simulink model "ICARO3_orientation_controllo_BIPE"  (R2014a)
settings: Solver=FixedStepDiscrete  SolverMode=MultiTasking  StartTime=0.0  StopTime=inf  FixedStep=0.001  RelTol=1e-3
PreLoadFcn:
  | Icaro_path;
  | 
  | load_param;
  | 
  | %override compute_alloc_inside load_param !!!
  | compute_alloc_esa;
  | 
  | load('mag_calib_sim_HIL.mat');
  | 
  | init_adaptive;
InitFcn:
  | %define fast control loop sample time
  | ST = 0.005;
  | 
  | %define filters
  | s = tf('s');
  | 
  | % Derivator (useful in PID controller)
  | D = 0.01*s/(0.01*s+1);
  | 
  | % LP 2nd order filter
  | LP = 42.88/(3.5*s^2 + 19.6*s + 42.88);
  | 
  | %load new DP position controllers
  | progetto_controllo_pos_v1;
undefined symbols (not defined in the file): DiscIntNeverNeededParam, Earth, G, H, INV_PITCH_RANGE, INV_ROLL_RANGE, INV_THROTTLE_RANGE, INV_YAW_RANGE, PITCH_IDX, PITCH_MID, ROLL_IDX, ROLL_MID, RTOL, THROTTLE_DOWN, THROTTLE_IDX, THROTTLE_LOW_THRES, Ts, WGS84, YAW_IDX, YAW_MID
libraries: simulink x15, GPIO_Lib x3, cstblocks x2, aerolibtransform2 x1, STM32_Config_Lib x1
(part 4 of 5)

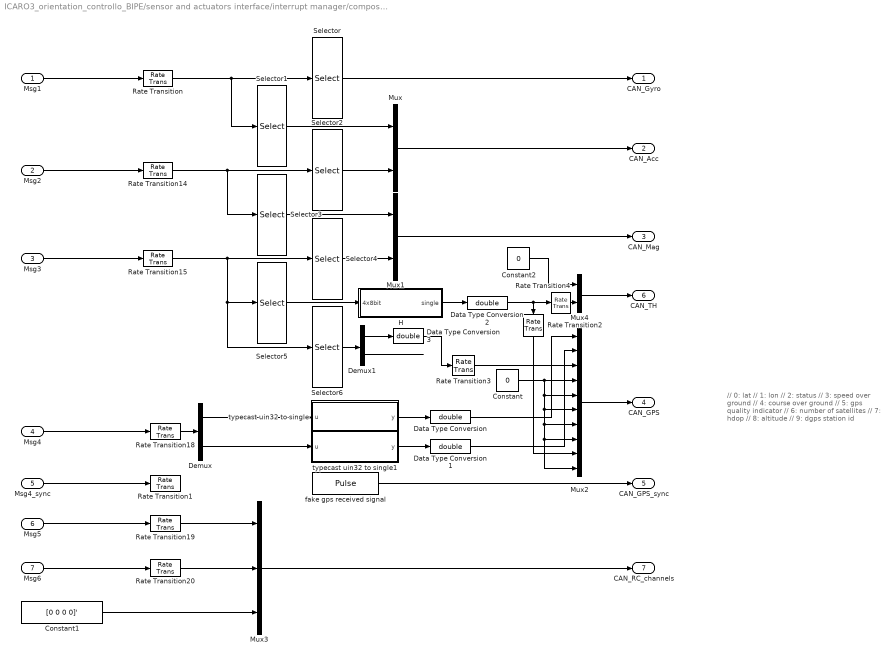
== system ICARO3_orientation_controllo_BIPE/sensor and actuators interface/interrupt manager/compose data from canbus ==
  note: // 0: lat
      |                         // 1: lon
      |                         // 2: status
      |                         // 3: speed over ground
      |                         // 4: course over ground
      |                         // 5: gps quality indicator
      |                         // 6: number of satellites
      |                         // 7: hdop
      |                         // 8: altitude
      |                         // 9: dgps station id
  Msg1 : Inport
  Msg2 : Inport  Port=2
  Msg3 : Inport  Port=3
  Msg4 : Inport  Port=4
  Msg4_sync : Inport  Port=5
  Msg5 : Inport  Port=6
  Msg6 : Inport  Port=7
  Constant : Constant  Value=0
  Constant1 : Constant  Value=[0 0 0 0]'  OutDataTypeStr=uint16
  Constant2 : Constant  Value=0
  Data Type Conversion{,1..3} (4 alike) : DataTypeConversion  OutDataTypeStr=double
  Demux : Demux  Outputs=2
  Demux1 : Demux  Outputs=2
  H : Subsystem
  Mux : Mux  Inputs=2
  Mux1 : Mux  Inputs=2
  Mux2 : Mux  Inputs=10
  Mux3 : Mux  Inputs=3
  Mux4 : Mux  Inputs=2
  Rate Transition{,1,14..15,18..20} (7 alike) : RateTransition  Deterministic=off
  Rate Transition2 : RateTransition
  Rate Transition3 : RateTransition
  Rate Transition4 : RateTransition
  Selector : Selector  InputPortWidth=8  Indices=[1:6]
  Selector1 : Selector  InputPortWidth=8  Indices=[7:8]
  Selector2 : Selector  InputPortWidth=8  Indices=[1:4]
  Selector3 : Selector  InputPortWidth=8  Indices=[5:8]
  Selector4 : Selector  InputPortWidth=8  Indices=[1:2]
  Selector5 : Selector  InputPortWidth=8  Indices=[3:6]
  Selector6 : Selector  InputPortWidth=8  Indices=[7:8]
  fake gps received signal : DiscretePulseGenerator  Period=20  SampleTime=0.01
  typecast uin32 to single : MATLAB Function  TreatAsAtomicUnit=on
      settings: RTWSystemCode=Inline
  typecast uin32 to single1 : MATLAB Function  TreatAsAtomicUnit=on
      settings: RTWSystemCode=Inline
  CAN_Gyro : Outport
  CAN_Acc : Outport  Port=2
  CAN_Mag : Outport  Port=3
  CAN_GPS : Outport  Port=4
  CAN_GPS_sync : Outport  Port=5
  CAN_TH : Outport  Port=6
  CAN_RC_channels : Outport  Port=7
  wires:
  typecast uin32 to single/1(y) -> Data Type Conversion/1
  Demux/1 -> typecast uin32 to single/1(u)
  Demux/2 -> typecast uin32 to single1/1(u)
  fake gps received signal/1 -> CAN_GPS_sync/1
  Data Type Conversion3/1 -> Rate Transition3/1
  Data Type Conversion2/1 -> Rate Transition4/1, Rate Transition2/1
  Data Type Conversion1/1 -> Mux2/2
  Data Type Conversion/1 -> Mux2/1
  Constant2/1 -> Mux4/1
  Rate Transition4/1 -> Mux4/2
  Rate Transition3/1 -> Mux2/3
  Rate Transition2/1 -> Mux2/9
  Mux4/1 -> CAN_TH/1
  Constant1/1 -> Mux3/3
  Mux3/1 -> CAN_RC_channels/1
  Mux2/1 -> CAN_GPS/1
  Demux1/2 -> ?
  Demux1/1 -> Data Type Conversion3/1
  Selector6/1 -> Demux1/1
  Constant/1 -> Mux2/10, Mux2/8, Mux2/7, Mux2/6, Mux2/5, Mux2/4
  Msg4_sync/1 -> Rate Transition1/1
  typecast uin32 to single1/1(y) -> Data Type Conversion1/1
  Rate Transition18/1 -> Demux/1
  H/1(single) -> Data Type Conversion2/1
  Selector5/1 -> H/1(4x8bit)
  Mux1/1 -> CAN_Mag/1
  Selector4/1 -> Mux1/2
  Rate Transition15/1 -> Selector6/1, Selector5/1, Selector4/1
  Selector3/1 -> Mux1/1
  Mux/1 -> CAN_Acc/1
  Selector1/1 -> Mux/1
  Selector2/1 -> Mux/2
  Rate Transition14/1 -> Selector3/1, Selector2/1
  Selector/1 -> CAN_Gyro/1
  Rate Transition/1 -> Selector1/1, Selector/1
  Rate Transition20/1 -> Mux3/2
  Msg6/1 -> Rate Transition20/1
  Rate Transition19/1 -> Mux3/1
  Msg5/1 -> Rate Transition19/1
  Msg4/1 -> Rate Transition18/1
  Msg3/1 -> Rate Transition15/1
  Msg2/1 -> Rate Transition14/1
  Msg1/1 -> Rate Transition/1

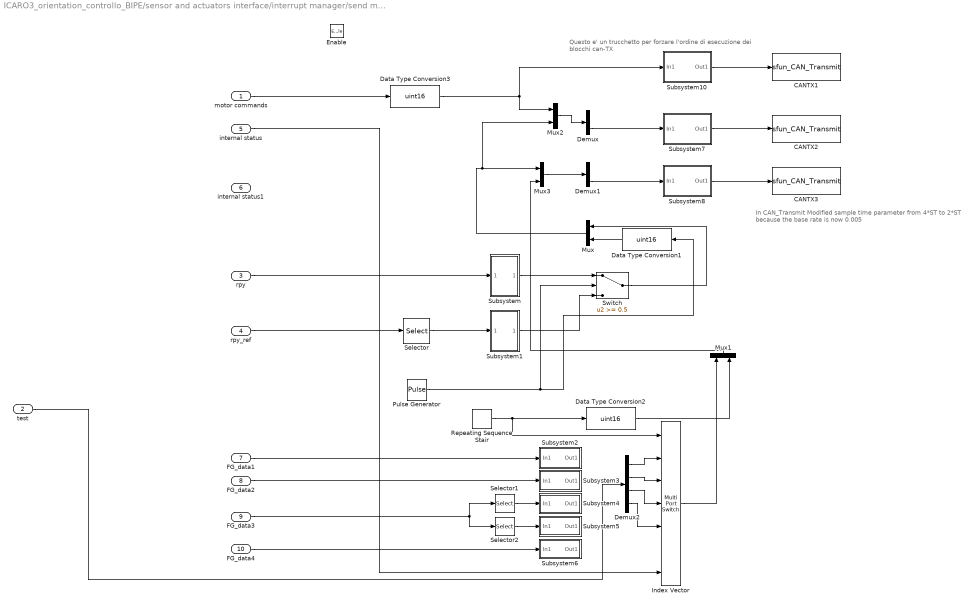
== system ICARO3_orientation_controllo_BIPE/sensor and actuators interface/interrupt manager/send motor commands via canbus ==
  note: In CAN_Transmit Modified sample time parameter from 4*ST to
      | 2*ST because the base rate is now 0.005
  note: Questo e' un trucchetto per forzare l'ordine di esecuzione
      | dei blocchi can-TX
  motor commands : Inport
  test : Inport  Port=2
  rpy : Inport  Port=3
  rpy_ref : Inport  Port=4
  internal status : Inport  Port=5
  internal status1 : Inport  Port=6
  FG_data1 : Inport  Port=7
  FG_data2 : Inport  Port=8
  FG_data3 : Inport  Port=9
  FG_data4 : Inport  Port=10
  Enable : EnablePort
  CANTX1 : S-Function  FunctionName=sfun_CAN_Transmit  Parameters=2*ST,bin2dec('10100001111'),8  EnableBusSupport=off
  CANTX2 : S-Function  FunctionName=sfun_CAN_Transmit  Parameters=2*ST,bin2dec('10100011111'),8  EnableBusSupport=off
  CANTX3 : S-Function  FunctionName=sfun_CAN_Transmit  Parameters=2*ST,bin2dec('10100101111'),8  EnableBusSupport=off
  Data Type Conversion1 : DataTypeConversion  OutDataTypeStr=uint16
  Data Type Conversion2 : DataTypeConversion  OutDataTypeStr=uint16  SampleTime=0.01
  Data Type Conversion3 : DataTypeConversion  OutDataTypeStr=uint16
  Demux : Demux  Outputs=[4 4]
  Demux1 : Demux  Outputs=[4 4]
  Demux2 : Demux  Outputs=[3 3 3 3]
  Index Vector : MultiPortSwitch  DataPortOrder=Zero-based contiguous  Inputs=6  zeroidx=on  SampleTime=0.01
  Mux{,1..3} (4 alike) : Mux  Inputs=2
  Pulse Generator : DiscretePulseGenerator  Period=4  PulseWidth=2  SampleTime=1/100
  Repeating Sequence Stair : simulink/Sources/Repeating Sequence Stair  OutValues=[0 0 1 1 2 2 3 3 4 4 5 5]  tsamp=0.01  OutMin=[]  OutMax=[]  OutDataTypeStr=double  OutputDataTypeScalingMode=double  OutDataType=fixdt(0,8)  ConRadixGroup=Best Precision: Vector-wise  OutScaling=2^-12
  Selector : Selector  InputPortWidth=4  Indices=2:4
  Selector1 : Selector  InputPortWidth=2
  Selector2 : Selector  InputPortWidth=2  Indices=2
  Subsystem : Subsystem
  Subsystem1 : Subsystem
  Subsystem10 : Subsystem
  Subsystem2 : Subsystem
  Subsystem3 : Subsystem
  Subsystem4 : Subsystem
  Subsystem5 : Subsystem
  Subsystem6 : Subsystem
  Subsystem7 : Subsystem
  Subsystem8 : Subsystem
  Switch : Switch  Threshold=0.5
  wires:
  Demux2/4 -> Index Vector/5
  Demux2/3 -> Index Vector/4
  Demux2/1 -> Index Vector/2
  Demux2/2 -> Index Vector/3
  Demux1/2 -> Subsystem8/1(In1)
  test/1 -> Demux2/1
  motor commands/1 -> Data Type Conversion3/1
  Subsystem8/1(Out1) -> CANTX3/1
  rpy_ref/1 -> Selector/1
  Subsystem1/1(Out1) -> Switch/3
  Demux/2 -> Subsystem7/1(In1)
  Subsystem7/1(Out1) -> CANTX2/1
  Subsystem10/1(Out1) -> CANTX1/1
  Data Type Conversion3/1 -> Mux2/1, Subsystem10/1(In1)
  Data Type Conversion2/1 -> Mux1/2
  Data Type Conversion1/1 -> Mux/2
  Repeating Sequence Stair/1 -> Index Vector/1, Data Type Conversion2/1
  FG_data4/1 -> Subsystem6/1(In1)
  FG_data3/1 -> Selector2/1, Selector1/1
  FG_data2/1 -> Subsystem3/1(In1)
  FG_data1/1 -> Subsystem2/1(In1)
  Selector2/1 -> Subsystem5/1(In1)
  Selector1/1 -> Subsystem4/1(In1)
  internal status/1 -> Index Vector/7
  Mux1/1 -> Mux3/2
  Mux3/1 -> Demux1/1
  Mux2/1 -> Demux/1
  Index Vector/1 -> Mux1/1
  Mux/1 -> Mux3/1, Mux2/2
  Selector/1 -> Subsystem1/1(In1)
  Pulse Generator/1 -> Data Type Conversion1/1, Switch/2
  Switch/1 -> Mux/1
  Subsystem/1(Out1) -> Switch/1
  rpy/1 -> Subsystem/1(In1)

== system ICARO3_orientation_controllo_BIPE/ADIS AHRS2/debias ADIS/Acceleration Detrend /Detrend ==
  Input : Inport
  Detrending : Inport  Port=2
  Constant1 : Constant  Value=0
  Subsystem : Subsystem  TreatAsAtomicUnit=on
  Sum1 : Sum  Inputs=|+-  SaturateOnIntegerOverflow=on  InputSameDT=on  OutDataTypeStr=Inherit: Same as first input
  Switch2 : Switch  Threshold=0.5  SaturateOnIntegerOverflow=on  InputSameDT=on
  Detrended Output : Outport
  wires:
  Sum1/1 -> Switch2/3
  Input/1 -> Subsystem/1(In1), Sum1/1
  Constant1/1 -> Switch2/1
  Subsystem/1(Out2) -> Sum1/2
  Detrending/1 -> Subsystem/Enable, Switch2/2
  Switch2/1 -> Detrended Output/1

== system ICARO3_orientation_controllo_BIPE/ADIS AHRS2/debias ADIS/Acceleration Detrend /Detrend1 ==
  Input : Inport
  Detrending : Inport  Port=2
  Constant1 : Constant  Value=0
  Subsystem : Subsystem  TreatAsAtomicUnit=on
  Sum1 : Sum  Inputs=|+-  SaturateOnIntegerOverflow=on  InputSameDT=on  OutDataTypeStr=Inherit: Same as first input
  Switch2 : Switch  Threshold=0.5  SaturateOnIntegerOverflow=on  InputSameDT=on
  Detrended Output : Outport
  wires:
  Switch2/1 -> Detrended Output/1
  Detrending/1 -> Switch2/2, Subsystem/Enable
  Subsystem/1(Out2) -> Sum1/2
  Constant1/1 -> Switch2/1
  Sum1/1 -> Switch2/3
  Input/1 -> Sum1/1, Subsystem/1(In1)

== system ICARO3_orientation_controllo_BIPE/ADIS AHRS2/debias ADIS/Acceleration Detrend /Detrend3 ==
  Input : Inport
  Detrending : Inport  Port=2
  Constant1 : Constant  Value=0
  Constant2 : Constant  Value=9.81
  Subsystem : Subsystem  TreatAsAtomicUnit=on
  Sum1 : Sum  Inputs=|+--  SaturateOnIntegerOverflow=on  InputSameDT=on  OutDataTypeStr=Inherit: Same as first input
  Switch2 : Switch  Threshold=0.5  SaturateOnIntegerOverflow=on  InputSameDT=on
  Detrended Output : Outport
  wires:
  Sum1/1 -> Switch2/3
  Constant2/1 -> Sum1/3
  Input/1 -> Subsystem/1(In1), Sum1/1
  Constant1/1 -> Switch2/1
  Subsystem/1(Out2) -> Sum1/2
  Detrending/1 -> Subsystem/Enable, Switch2/2
  Switch2/1 -> Detrended Output/1

== system ICARO3_orientation_controllo_BIPE/ADIS AHRS2/debias ADIS/Gyros Detrend/Detrend ==
  Input : Inport
  Detrending : Inport  Port=2
  Constant1 : Constant  Value=0
  Subsystem : Subsystem  TreatAsAtomicUnit=on
  Sum1 : Sum  Inputs=|+-  SaturateOnIntegerOverflow=on  InputSameDT=on  OutDataTypeStr=Inherit: Same as first input
  Switch2 : Switch  Threshold=0.5  SaturateOnIntegerOverflow=on  InputSameDT=on
  Detrended Output : Outport
  wires:
  Sum1/1 -> Switch2/3
  Switch2/1 -> Detrended Output/1
  Detrending/1 -> Switch2/2, Subsystem/Enable
  Subsystem/1(Out2) -> Sum1/2
  Constant1/1 -> Switch2/1
  Input/1 -> Sum1/1, Subsystem/1(In1)

== system ICARO3_orientation_controllo_BIPE/ADIS AHRS2/debias ADIS/Gyros Detrend/Detrend1 ==
  Input : Inport
  Detrending : Inport  Port=2
  Constant1 : Constant  Value=0
  Subsystem : Subsystem  TreatAsAtomicUnit=on
  Sum1 : Sum  Inputs=|+-  SaturateOnIntegerOverflow=on  InputSameDT=on  OutDataTypeStr=Inherit: Same as first input
  Switch2 : Switch  Threshold=0.5  SaturateOnIntegerOverflow=on  InputSameDT=on
  Detrended Output : Outport
  wires:
  Sum1/1 -> Switch2/3
  Input/1 -> Subsystem/1(In1), Sum1/1
  Constant1/1 -> Switch2/1
  Subsystem/1(Out2) -> Sum1/2
  Detrending/1 -> Subsystem/Enable, Switch2/2
  Switch2/1 -> Detrended Output/1

== system ICARO3_orientation_controllo_BIPE/ADIS AHRS2/debias ADIS/Gyros Detrend/Detrend2 ==
  Input : Inport
  Detrending : Inport  Port=2
  Constant1 : Constant  Value=0
  Subsystem : Subsystem  TreatAsAtomicUnit=on
  Sum1 : Sum  Inputs=|+-  SaturateOnIntegerOverflow=on  InputSameDT=on  OutDataTypeStr=Inherit: Same as first input
  Switch2 : Switch  Threshold=0.5  SaturateOnIntegerOverflow=on  InputSameDT=on
  Detrended Output : Outport
  wires:
  Sum1/1 -> Switch2/3
  Switch2/1 -> Detrended Output/1
  Detrending/1 -> Switch2/2, Subsystem/Enable
  Subsystem/1(Out2) -> Sum1/2
  Constant1/1 -> Switch2/1
  Input/1 -> Sum1/1, Subsystem/1(In1)

== system ICARO3_orientation_controllo_BIPE/ADIS AHRS2/debias ADIS1/Acceleration Detrend /Detrend ==
  Input : Inport
  Detrending : Inport  Port=2
  Constant1 : Constant  Value=0  OutDataTypeStr=single
  Subsystem : Subsystem  TreatAsAtomicUnit=on
  Sum1 : Sum  Inputs=|+-  SaturateOnIntegerOverflow=on  InputSameDT=on  OutDataTypeStr=Inherit: Same as first input
  Switch2 : Switch  Threshold=0.5  SaturateOnIntegerOverflow=on  InputSameDT=on
  Detrended Output : Outport
  wires:
  Sum1/1 -> Switch2/3
  Input/1 -> Subsystem/1(In1), Sum1/1
  Constant1/1 -> Switch2/1
  Subsystem/1(Out2) -> Sum1/2
  Detrending/1 -> Subsystem/Enable, Switch2/2
  Switch2/1 -> Detrended Output/1

== system ICARO3_orientation_controllo_BIPE/ADIS AHRS2/debias ADIS1/Acceleration Detrend /Detrend1 ==
  Input : Inport
  Detrending : Inport  Port=2
  Constant1 : Constant  Value=0  OutDataTypeStr=single
  Subsystem : Subsystem  TreatAsAtomicUnit=on
  Sum1 : Sum  Inputs=|+-  SaturateOnIntegerOverflow=on  InputSameDT=on  OutDataTypeStr=Inherit: Same as first input
  Switch2 : Switch  Threshold=0.5  SaturateOnIntegerOverflow=on  InputSameDT=on
  Detrended Output : Outport
  wires:
  Switch2/1 -> Detrended Output/1
  Detrending/1 -> Switch2/2, Subsystem/Enable
  Subsystem/1(Out2) -> Sum1/2
  Constant1/1 -> Switch2/1
  Sum1/1 -> Switch2/3
  Input/1 -> Sum1/1, Subsystem/1(In1)

== system ICARO3_orientation_controllo_BIPE/ADIS AHRS2/debias ADIS1/Acceleration Detrend /Detrend3 ==
  Input : Inport
  Detrending : Inport  Port=2
  Constant1 : Constant  Value=0  OutDataTypeStr=single
  Constant2 : Constant  Value=9.81  OutDataTypeStr=single
  Subsystem : Subsystem  TreatAsAtomicUnit=on
  Sum1 : Sum  Inputs=|+--  SaturateOnIntegerOverflow=on  InputSameDT=on  OutDataTypeStr=Inherit: Same as first input
  Switch2 : Switch  Threshold=0.5  SaturateOnIntegerOverflow=on  InputSameDT=on
  Detrended Output : Outport
  wires:
  Sum1/1 -> Switch2/3
  Constant2/1 -> Sum1/3
  Input/1 -> Subsystem/1(In1), Sum1/1
  Constant1/1 -> Switch2/1
  Subsystem/1(Out2) -> Sum1/2
  Switch2/1 -> Detrended Output/1
  Detrending/1 -> Switch2/2, Subsystem/Enable

== system ICARO3_orientation_controllo_BIPE/ADIS AHRS2/debias ADIS1/Acceleration Detrend 1/Detrend ==
  Input : Inport
  Detrending : Inport  Port=2
  Constant1 : Constant  Value=0
  Subsystem : Subsystem  TreatAsAtomicUnit=on
  Sum1 : Sum  Inputs=|+-  SaturateOnIntegerOverflow=on  InputSameDT=on  OutDataTypeStr=Inherit: Same as first input
  Switch2 : Switch  Threshold=0.5  SaturateOnIntegerOverflow=on  InputSameDT=on
  Detrended Output : Outport
  wires:
  Sum1/1 -> Switch2/3
  Input/1 -> Subsystem/1(In1), Sum1/1
  Constant1/1 -> Switch2/1
  Subsystem/1(Out2) -> Sum1/2
  Detrending/1 -> Subsystem/Enable, Switch2/2
  Switch2/1 -> Detrended Output/1

== system ICARO3_orientation_controllo_BIPE/ADIS AHRS2/debias ADIS1/Acceleration Detrend 1/Detrend1 ==
  Input : Inport
  Detrending : Inport  Port=2
  Constant1 : Constant  Value=0
  Subsystem : Subsystem  TreatAsAtomicUnit=on
  Sum1 : Sum  Inputs=|+-  SaturateOnIntegerOverflow=on  InputSameDT=on  OutDataTypeStr=Inherit: Same as first input
  Switch2 : Switch  Threshold=0.5  SaturateOnIntegerOverflow=on  InputSameDT=on
  Detrended Output : Outport
  wires:
  Switch2/1 -> Detrended Output/1
  Detrending/1 -> Switch2/2, Subsystem/Enable
  Subsystem/1(Out2) -> Sum1/2
  Constant1/1 -> Switch2/1
  Sum1/1 -> Switch2/3
  Input/1 -> Sum1/1, Subsystem/1(In1)

== system ICARO3_orientation_controllo_BIPE/ADIS AHRS2/debias ADIS1/Acceleration Detrend 1/Detrend3 ==
  Input : Inport
  Detrending : Inport  Port=2  OutDataTypeStr=single
  Constant1 : Constant  Value=0
  Constant2 : Constant  Value=9.81
  Subsystem : Subsystem  TreatAsAtomicUnit=on
  Sum1 : Sum  Inputs=|+--  SaturateOnIntegerOverflow=on  InputSameDT=on  OutDataTypeStr=Inherit: Same as first input
  Switch2 : Switch  Threshold=0.5  SaturateOnIntegerOverflow=on  InputSameDT=on
  Detrended Output : Outport
  wires:
  Sum1/1 -> Switch2/3
  Constant2/1 -> Sum1/3
  Input/1 -> Subsystem/1(In1), Sum1/1
  Constant1/1 -> Switch2/1
  Subsystem/1(Out2) -> Sum1/2
  Switch2/1 -> Detrended Output/1
  Detrending/1 -> Switch2/2, Subsystem/Enable

== system ICARO3_orientation_controllo_BIPE/ADIS AHRS2/debias ADIS1/Gyros Detrend/Detrend ==
  Input : Inport
  Detrending : Inport  Port=2
  Constant1 : Constant  Value=0
  Data Type Conversion mx3 : DataTypeConversion  OutDataTypeStr=double  RndMeth=Round  SaturateOnIntegerOverflow=on
  Subsystem : Subsystem  TreatAsAtomicUnit=on
  Sum1 : Sum  Inputs=|+-  SaturateOnIntegerOverflow=on  InputSameDT=on  OutDataTypeStr=Inherit: Same as first input
  Switch2 : Switch  Threshold=0.5  SaturateOnIntegerOverflow=on  InputSameDT=on
  Detrended Output : Outport
  wires:
  Switch2/1 -> Detrended Output/1
  Detrending/1 -> Switch2/2, Subsystem/Enable
  Subsystem/1(Out2) -> Sum1/2
  Constant1/1 -> Switch2/1
  Input/1 -> Sum1/1, Subsystem/1(In1)
  Sum1/1 -> Data Type Conversion mx3/1
  Data Type Conversion mx3/1 -> Switch2/3

== system ICARO3_orientation_controllo_BIPE/ADIS AHRS2/debias ADIS1/Gyros Detrend/Detrend1 ==
  Input : Inport
  Detrending : Inport  Port=2
  Constant1 : Constant  Value=0
  Data Type Conversion mx3 : DataTypeConversion  OutDataTypeStr=double  RndMeth=Round  SaturateOnIntegerOverflow=on
  Subsystem : Subsystem  TreatAsAtomicUnit=on
  Sum1 : Sum  Inputs=|+-  SaturateOnIntegerOverflow=on  InputSameDT=on  OutDataTypeStr=Inherit: Same as first input
  Switch2 : Switch  Threshold=0.5  SaturateOnIntegerOverflow=on  InputSameDT=on
  Detrended Output : Outport
  wires:
  Sum1/1 -> Data Type Conversion mx3/1
  Input/1 -> Subsystem/1(In1), Sum1/1
  Constant1/1 -> Switch2/1
  Subsystem/1(Out2) -> Sum1/2
  Detrending/1 -> Subsystem/Enable, Switch2/2
  Switch2/1 -> Detrended Output/1
  Data Type Conversion mx3/1 -> Switch2/3

== system ICARO3_orientation_controllo_BIPE/ADIS AHRS2/debias ADIS1/Gyros Detrend/Detrend2 ==
  Input : Inport
  Detrending : Inport  Port=2
  Constant1 : Constant  Value=0
  Data Type Conversion mx3 : DataTypeConversion  OutDataTypeStr=double  RndMeth=Round  SaturateOnIntegerOverflow=on
  Subsystem : Subsystem  TreatAsAtomicUnit=on
  Sum1 : Sum  Inputs=|+-  SaturateOnIntegerOverflow=on  InputSameDT=on  OutDataTypeStr=Inherit: Same as first input
  Switch2 : Switch  Threshold=0.5  SaturateOnIntegerOverflow=on  InputSameDT=on
  Detrended Output : Outport
  wires:
  Sum1/1 -> Data Type Conversion mx3/1
  Switch2/1 -> Detrended Output/1
  Detrending/1 -> Switch2/2, Subsystem/Enable
  Subsystem/1(Out2) -> Sum1/2
  Constant1/1 -> Switch2/1
  Input/1 -> Sum1/1, Subsystem/1(In1)
  Data Type Conversion mx3/1 -> Switch2/3

== system ICARO3_orientation_controllo_BIPE/SS AHRS/debias SS/Acceleration Detrend /Detrend ==
  Input : Inport
  Detrending : Inport  Port=2
  Constant1 : Constant  Value=0
  Subsystem : Subsystem  TreatAsAtomicUnit=on
  Sum1 : Sum  Inputs=|+-  SaturateOnIntegerOverflow=on  InputSameDT=on  OutDataTypeStr=Inherit: Same as first input
  Switch2 : Switch  Threshold=0.5  SaturateOnIntegerOverflow=on  InputSameDT=on
  Detrended Output : Outport
  wires:
  Switch2/1 -> Detrended Output/1
  Detrending/1 -> Switch2/2, Subsystem/Enable
  Subsystem/1(Out2) -> Sum1/2
  Constant1/1 -> Switch2/1
  Input/1 -> Sum1/1, Subsystem/1(In1)
  Sum1/1 -> Switch2/3

== system ICARO3_orientation_controllo_BIPE/SS AHRS/debias SS/Acceleration Detrend /Detrend1 ==
  Input : Inport
  Detrending : Inport  Port=2
  Constant1 : Constant  Value=0
  Subsystem : Subsystem  TreatAsAtomicUnit=on
  Sum1 : Sum  Inputs=|+-  SaturateOnIntegerOverflow=on  InputSameDT=on  OutDataTypeStr=Inherit: Same as first input
  Switch2 : Switch  Threshold=0.5  SaturateOnIntegerOverflow=on  InputSameDT=on
  Detrended Output : Outport
  wires:
  Input/1 -> Subsystem/1(In1), Sum1/1
  Sum1/1 -> Switch2/3
  Constant1/1 -> Switch2/1
  Subsystem/1(Out2) -> Sum1/2
  Detrending/1 -> Subsystem/Enable, Switch2/2
  Switch2/1 -> Detrended Output/1

== system ICARO3_orientation_controllo_BIPE/SS AHRS/debias SS/Acceleration Detrend /Detrend3 ==
  Input : Inport
  Detrending : Inport  Port=2
  Constant1 : Constant  Value=0
  Constant2 : Constant  Value=9.81
  Subsystem : Subsystem  TreatAsAtomicUnit=on
  Sum1 : Sum  Inputs=|+--  SaturateOnIntegerOverflow=on  InputSameDT=on  OutDataTypeStr=Inherit: Same as first input
  Switch2 : Switch  Threshold=0.5  SaturateOnIntegerOverflow=on  InputSameDT=on
  Detrended Output : Outport
  wires:
  Switch2/1 -> Detrended Output/1
  Detrending/1 -> Switch2/2, Subsystem/Enable
  Subsystem/1(Out2) -> Sum1/2
  Constant1/1 -> Switch2/1
  Input/1 -> Sum1/1, Subsystem/1(In1)
  Constant2/1 -> Sum1/3
  Sum1/1 -> Switch2/3

== system ICARO3_orientation_controllo_BIPE/SS AHRS/debias SS/Gyros Detrend/Detrend ==
  Input : Inport
  Detrending : Inport  Port=2
  Constant1 : Constant  Value=0
  Subsystem : Subsystem  TreatAsAtomicUnit=on
  Sum1 : Sum  Inputs=|+-  SaturateOnIntegerOverflow=on  InputSameDT=on  OutDataTypeStr=Inherit: Same as first input
  Switch2 : Switch  Threshold=0.5  SaturateOnIntegerOverflow=on  InputSameDT=on
  Detrended Output : Outport
  wires:
  Input/1 -> Subsystem/1(In1), Sum1/1
  Constant1/1 -> Switch2/1
  Subsystem/1(Out2) -> Sum1/2
  Detrending/1 -> Subsystem/Enable, Switch2/2
  Switch2/1 -> Detrended Output/1
  Sum1/1 -> Switch2/3

== system ICARO3_orientation_controllo_BIPE/SS AHRS/debias SS/Gyros Detrend/Detrend1 ==
  Input : Inport
  Detrending : Inport  Port=2
  Constant1 : Constant  Value=0
  Subsystem : Subsystem  TreatAsAtomicUnit=on
  Sum1 : Sum  Inputs=|+-  SaturateOnIntegerOverflow=on  InputSameDT=on  OutDataTypeStr=Inherit: Same as first input
  Switch2 : Switch  Threshold=0.5  SaturateOnIntegerOverflow=on  InputSameDT=on
  Detrended Output : Outport
  wires:
  Switch2/1 -> Detrended Output/1
  Detrending/1 -> Switch2/2, Subsystem/Enable
  Subsystem/1(Out2) -> Sum1/2
  Constant1/1 -> Switch2/1
  Input/1 -> Sum1/1, Subsystem/1(In1)
  Sum1/1 -> Switch2/3

== system ICARO3_orientation_controllo_BIPE/SS AHRS/debias SS/Gyros Detrend/Detrend2 ==
  Input : Inport
  Detrending : Inport  Port=2
  Constant1 : Constant  Value=0
  Subsystem : Subsystem  TreatAsAtomicUnit=on
  Sum1 : Sum  Inputs=|+-  SaturateOnIntegerOverflow=on  InputSameDT=on  OutDataTypeStr=Inherit: Same as first input
  Switch2 : Switch  Threshold=0.5  SaturateOnIntegerOverflow=on  InputSameDT=on
  Detrended Output : Outport
  wires:
  Input/1 -> Subsystem/1(In1), Sum1/1
  Constant1/1 -> Switch2/1
  Subsystem/1(Out2) -> Sum1/2
  Detrending/1 -> Subsystem/Enable, Switch2/2
  Switch2/1 -> Detrended Output/1
  Sum1/1 -> Switch2/3

== system ICARO3_orientation_controllo_BIPE/sensor and actuators interface/interrupt manager/Arrange pwms/clock latch ==
  note: NOTE: initial output value of OUTPORT
      | is set to -1000 to ensure that the first computed age
      | at the start of autopilot is at least 1000 !
      | (otherwise it was 0)
  In : Inport
  Enable : EnablePort
  Out : Outport  InitialOutput=-1000
  wires:
  In/1 -> Out/1

== system ICARO3_orientation_controllo_BIPE/sensor and actuators interface/interrupt manager/CANbus data RX/Subsystem1 ==
  In1 : Inport
  Data Type Conversion on i2c mag1 : DataTypeConversion  OutDataTypeStr=uint16
  Demux3 : Demux  Outputs=[ 2 2 2 2]
  MATLAB Function compute gyroxyz1 : MATLAB Function  TreatAsAtomicUnit=on
  MATLAB Function compute gyroxyz2 : MATLAB Function  TreatAsAtomicUnit=on
  MATLAB Function compute gyroxyz3 : MATLAB Function  TreatAsAtomicUnit=on
  MATLAB Function compute gyroxyz5 : MATLAB Function  TreatAsAtomicUnit=on
  Mux : Mux
  Out1 : Outport
  wires:
  MATLAB Function compute gyroxyz5/1(y) -> Mux/1
  Mux/1 -> Out1/1
  MATLAB Function compute gyroxyz3/1(y) -> Mux/4
  MATLAB Function compute gyroxyz1/1(y) -> Mux/2
  Demux3/2 -> MATLAB Function compute gyroxyz1/1(u)
  Demux3/3 -> MATLAB Function compute gyroxyz2/1(u)
  MATLAB Function compute gyroxyz2/1(y) -> Mux/3
  Data Type Conversion on i2c mag1/1 -> Demux3/1
  Demux3/1 -> MATLAB Function compute gyroxyz5/1(u)
  In1/1 -> Data Type Conversion on i2c mag1/1
  Demux3/4 -> MATLAB Function compute gyroxyz3/1(u)

== system ICARO3_orientation_controllo_BIPE/sensor and actuators interface/interrupt manager/CANbus data RX/Subsystem2 ==
  In1 : Inport
  Data Type Conversion on i2c mag1 : DataTypeConversion  OutDataTypeStr=uint32
  Demux3 : Demux  Outputs=[ 4 4]
  MATLAB Function compute gyroxyz1 : MATLAB Function  TreatAsAtomicUnit=on
  MATLAB Function compute gyroxyz5 : MATLAB Function  TreatAsAtomicUnit=on
  Mux : Mux  Inputs=2
  Out1 : Outport
  wires:
  MATLAB Function compute gyroxyz1/1(y) -> Mux/2
  Demux3/2 -> MATLAB Function compute gyroxyz1/1(u)
  Data Type Conversion on i2c mag1/1 -> Demux3/1
  MATLAB Function compute gyroxyz5/1(y) -> Mux/1
  Demux3/1 -> MATLAB Function compute gyroxyz5/1(u)
  In1/1 -> Data Type Conversion on i2c mag1/1
  Mux/1 -> Out1/1

== system ICARO3_orientation_controllo_BIPE/sensor and actuators interface/interrupt manager/CANbus data RX/Subsystem3 ==
  In1 : Inport
  Data Type Conversion on i2c mag1 : DataTypeConversion  OutDataTypeStr=uint16
  Demux3 : Demux  Outputs=[ 2 2 2 2]
  MATLAB Function compute gyroxyz1 : MATLAB Function  TreatAsAtomicUnit=on
  MATLAB Function compute gyroxyz2 : MATLAB Function  TreatAsAtomicUnit=on
  MATLAB Function compute gyroxyz3 : MATLAB Function  TreatAsAtomicUnit=on
  MATLAB Function compute gyroxyz5 : MATLAB Function  TreatAsAtomicUnit=on
  Mux : Mux
  Out1 : Outport
  wires:
  Demux3/4 -> MATLAB Function compute gyroxyz3/1(u)
  In1/1 -> Data Type Conversion on i2c mag1/1
  Demux3/1 -> MATLAB Function compute gyroxyz5/1(u)
  Data Type Conversion on i2c mag1/1 -> Demux3/1
  MATLAB Function compute gyroxyz2/1(y) -> Mux/3
  Demux3/3 -> MATLAB Function compute gyroxyz2/1(u)
  Demux3/2 -> MATLAB Function compute gyroxyz1/1(u)
  MATLAB Function compute gyroxyz1/1(y) -> Mux/2
  MATLAB Function compute gyroxyz3/1(y) -> Mux/4
  Mux/1 -> Out1/1
  MATLAB Function compute gyroxyz5/1(y) -> Mux/1

== matlab function ICARO3_orientation_controllo_BIPE/sensor and actuators interface/interrupt manager/send motor commands via canbus/Subsystem7/MATLAB Function compute gyroxyz1 ==
  settings: updateMethod=DISCRETE  sampleTime=0.01
  data: u input uint16; y output uint8
function y = pack2_8bit(u)

y =uint8([0,0]);
y(1) = bitand(u,255);
y(2) = bitshift(u,-8);

== matlab function ICARO3_orientation_controllo_BIPE/sensor and actuators interface/interrupt manager/send motor commands via canbus/Subsystem7/MATLAB Function compute gyroxyz4 ==
  settings: updateMethod=DISCRETE  sampleTime=0.01
  data: u input uint8; y output uint8
function y = reorder(u)

y=uint8(zeros(1,8));
y(1)=u(1);
y(2)=u(2);
y(3)=u(3);
y(4)=u(4);
y(5)=u(5);
y(6)=u(6);
y(7)=u(7);
y(8)=u(8);

== matlab function ICARO3_orientation_controllo_BIPE/sensor and actuators interface/interrupt manager/send motor commands via canbus/Subsystem8/MATLAB Function compute gyroxyz4 ==
  settings: updateMethod=DISCRETE  sampleTime=0.01
  data: u input uint8; y output uint8
function y = reorder(u)

y=uint8(zeros(1,8));
y(1)=u(1);
y(2)=u(2);
y(3)=u(3);
y(4)=u(4);
y(5)=u(5);
y(6)=u(6);
y(7)=u(7);
y(8)=u(8);

== system ICARO3_orientation_controllo_BIPE/sensor and actuators interface/interrupt manager/compose data from canbus/H ==
  4x8bit : Inport
  " " : ArithShift  BitShiftNumber=24  BitShiftDirection=Left
  "  " : ArithShift  BitShiftNumber=16  BitShiftDirection=Left
  "  2" : ArithShift  BitShiftNumber=8  BitShiftDirection=Left
  Data Type Conversion{7..10} (4 alike) : DataTypeConversion  OutDataTypeStr=uint32
  Demux : Demux
  Sum12 : Sum  Inputs=++++
  typecast uin32 to single : MATLAB Function  TreatAsAtomicUnit=on
      settings: RTWSystemCode=Inline
  single : Outport
  wires:
  4x8bit/1 -> Demux/1
  Demux/4 -> Data Type Conversion10/1
  Demux/3 -> Data Type Conversion7/1
  Demux/2 -> Data Type Conversion9/1
  Demux/1 -> Data Type Conversion8/1
  typecast uin32 to single/1(y) -> single/1
  Sum12/1 -> typecast uin32 to single/1(u)
  " "/1 -> Sum12/1
  Data Type Conversion10/1 -> Sum12/4
  "  2"/1 -> Sum12/3
  "  "/1 -> Sum12/2
  Data Type Conversion7/1 -> "  2"/1
  Data Type Conversion9/1 -> "  "/1
  Data Type Conversion8/1 -> " "/1

== system ICARO3_orientation_controllo_BIPE/sensor and actuators interface/interrupt manager/send motor commands via canbus/Subsystem ==
  In1 : Inport
  Constant : Constant  Value=180
  Data Type Conversion2 : DataTypeConversion  OutDataTypeStr=uint16
  Gain : Gain  Gain=180/pi
  Sum : Sum  Inputs=|++
  Out1 : Outport
  wires:
  In1/1 -> Gain/1
  Data Type Conversion2/1 -> Out1/1
  Sum/1 -> Data Type Conversion2/1
  Constant/1 -> Sum/2
  Gain/1 -> Sum/1

== system ICARO3_orientation_controllo_BIPE/sensor and actuators interface/interrupt manager/send motor commands via canbus/Subsystem1 ==
  In1 : Inport
  Constant : Constant  Value=180
  Data Type Conversion2 : DataTypeConversion  OutDataTypeStr=uint16
  Gain : Gain  Gain=180/pi
  Sum : Sum  Inputs=|++
  Out1 : Outport
  wires:
  Gain/1 -> Sum/1
  Constant/1 -> Sum/2
  Sum/1 -> Data Type Conversion2/1
  Data Type Conversion2/1 -> Out1/1
  In1/1 -> Gain/1

== system ICARO3_orientation_controllo_BIPE/sensor and actuators interface/interrupt manager/send motor commands via canbus/Subsystem10 ==
  In1 : Inport
  Demux3 : Demux  Outputs=[1 1 1 1]
  MATLAB Function compute gyroxyz1 : MATLAB Function  TreatAsAtomicUnit=on
  MATLAB Function compute gyroxyz2 : MATLAB Function  TreatAsAtomicUnit=on
  MATLAB Function compute gyroxyz3 : MATLAB Function  TreatAsAtomicUnit=on
  MATLAB Function compute gyroxyz4 : MATLAB Function  TreatAsAtomicUnit=on
  MATLAB Function compute gyroxyz5 : MATLAB Function  TreatAsAtomicUnit=on
  Mux1 : Mux  Inputs=[2 2 2 2]
  Out1 : Outport
  wires:
  MATLAB Function compute gyroxyz4/1(y) -> Out1/1
  Mux1/1 -> MATLAB Function compute gyroxyz4/1(u)
  MATLAB Function compute gyroxyz5/1(y) -> Mux1/1
  MATLAB Function compute gyroxyz3/1(y) -> Mux1/4
  MATLAB Function compute gyroxyz2/1(y) -> Mux1/3
  MATLAB Function compute gyroxyz1/1(y) -> Mux1/2
  Demux3/2 -> MATLAB Function compute gyroxyz1/1(u)
  Demux3/3 -> MATLAB Function compute gyroxyz2/1(u)
  In1/1 -> Demux3/1
  Demux3/1 -> MATLAB Function compute gyroxyz5/1(u)
  Demux3/4 -> MATLAB Function compute gyroxyz3/1(u)

== system ICARO3_orientation_controllo_BIPE/sensor and actuators interface/interrupt manager/send motor commands via canbus/Subsystem2 ==
  In1 : Inport
  Constant : Constant  Value=2047  SampleTime=0.01
  Data Type Conversion2 : DataTypeConversion  OutDataTypeStr=uint16
  Gain : Gain  Gain=100
  Sum : Sum  Inputs=|++
  Out1 : Outport
  wires:
  Gain/1 -> Sum/1
  Constant/1 -> Sum/2
  Sum/1 -> Data Type Conversion2/1
  Data Type Conversion2/1 -> Out1/1
  In1/1 -> Gain/1

== system ICARO3_orientation_controllo_BIPE/sensor and actuators interface/interrupt manager/send motor commands via canbus/Subsystem3 ==
  In1 : Inport
  Constant : Constant  Value=2047  SampleTime=0.01
  Data Type Conversion2 : DataTypeConversion  OutDataTypeStr=uint16
  Gain : Gain  Gain=100
  Sum : Sum  Inputs=|++
  Out1 : Outport
  wires:
  In1/1 -> Gain/1
  Data Type Conversion2/1 -> Out1/1
  Sum/1 -> Data Type Conversion2/1
  Constant/1 -> Sum/2
  Gain/1 -> Sum/1

== system ICARO3_orientation_controllo_BIPE/sensor and actuators interface/interrupt manager/send motor commands via canbus/Subsystem4 ==
  In1 : Inport
  Constant : Constant  Value=2047  SampleTime=0.01
  Data Type Conversion2 : DataTypeConversion  OutDataTypeStr=uint16
  Gain : Gain  Gain=100
  Sum : Sum  Inputs=|++
  Out1 : Outport
  wires:
  Gain/1 -> Sum/1
  Constant/1 -> Sum/2
  Sum/1 -> Data Type Conversion2/1
  Data Type Conversion2/1 -> Out1/1
  In1/1 -> Gain/1

== system ICARO3_orientation_controllo_BIPE/sensor and actuators interface/interrupt manager/send motor commands via canbus/Subsystem5 ==
  In1 : Inport
  Constant : Constant  Value=2047  SampleTime=0.01
  Data Type Conversion2 : DataTypeConversion  OutDataTypeStr=uint16
  Gain : Gain  Gain=100
  Sum : Sum  Inputs=|++
  Out1 : Outport
  wires:
  In1/1 -> Gain/1
  Data Type Conversion2/1 -> Out1/1
  Sum/1 -> Data Type Conversion2/1
  Constant/1 -> Sum/2
  Gain/1 -> Sum/1

== system ICARO3_orientation_controllo_BIPE/sensor and actuators interface/interrupt manager/send motor commands via canbus/Subsystem6 ==
  In1 : Inport
  Constant : Constant  Value=2047  SampleTime=0.01
  Data Type Conversion2 : DataTypeConversion  OutDataTypeStr=uint16
  Gain : Gain  Gain=100
  Sum : Sum  Inputs=|++
  Out1 : Outport
  wires:
  Gain/1 -> Sum/1
  Constant/1 -> Sum/2
  Sum/1 -> Data Type Conversion2/1
  Data Type Conversion2/1 -> Out1/1
  In1/1 -> Gain/1

== system ICARO3_orientation_controllo_BIPE/sensor and actuators interface/interrupt manager/send motor commands via canbus/Subsystem7 ==
  In1 : Inport
  Demux3 : Demux  Outputs=[1 1 1 1]
  MATLAB Function compute gyroxyz1 : MATLAB Function  TreatAsAtomicUnit=on
  MATLAB Function compute gyroxyz2 : MATLAB Function  TreatAsAtomicUnit=on
  MATLAB Function compute gyroxyz3 : MATLAB Function  TreatAsAtomicUnit=on
  MATLAB Function compute gyroxyz4 : MATLAB Function  TreatAsAtomicUnit=on
  MATLAB Function compute gyroxyz5 : MATLAB Function  TreatAsAtomicUnit=on
  Mux1 : Mux  Inputs=[2 2 2 2]
  Out1 : Outport
  wires:
  Demux3/4 -> MATLAB Function compute gyroxyz3/1(u)
  Demux3/1 -> MATLAB Function compute gyroxyz5/1(u)
  In1/1 -> Demux3/1
  Demux3/3 -> MATLAB Function compute gyroxyz2/1(u)
  Demux3/2 -> MATLAB Function compute gyroxyz1/1(u)
  MATLAB Function compute gyroxyz1/1(y) -> Mux1/2
  MATLAB Function compute gyroxyz2/1(y) -> Mux1/3
  MATLAB Function compute gyroxyz3/1(y) -> Mux1/4
  MATLAB Function compute gyroxyz5/1(y) -> Mux1/1
  Mux1/1 -> MATLAB Function compute gyroxyz4/1(u)
  MATLAB Function compute gyroxyz4/1(y) -> Out1/1

== system ICARO3_orientation_controllo_BIPE/sensor and actuators interface/interrupt manager/send motor commands via canbus/Subsystem8 ==
  In1 : Inport
  Demux3 : Demux  Outputs=[1 1 1 1]
  MATLAB Function compute gyroxyz1 : MATLAB Function  TreatAsAtomicUnit=on
  MATLAB Function compute gyroxyz2 : MATLAB Function  TreatAsAtomicUnit=on
  MATLAB Function compute gyroxyz3 : MATLAB Function  TreatAsAtomicUnit=on
  MATLAB Function compute gyroxyz4 : MATLAB Function  TreatAsAtomicUnit=on
  MATLAB Function compute gyroxyz5 : MATLAB Function  TreatAsAtomicUnit=on
  Mux1 : Mux  Inputs=[2 2 2 2]
  Out1 : Outport
  wires:
  MATLAB Function compute gyroxyz4/1(y) -> Out1/1
  Mux1/1 -> MATLAB Function compute gyroxyz4/1(u)
  MATLAB Function compute gyroxyz5/1(y) -> Mux1/1
  MATLAB Function compute gyroxyz3/1(y) -> Mux1/4
  MATLAB Function compute gyroxyz2/1(y) -> Mux1/3
  MATLAB Function compute gyroxyz1/1(y) -> Mux1/2
  Demux3/2 -> MATLAB Function compute gyroxyz1/1(u)
  Demux3/3 -> MATLAB Function compute gyroxyz2/1(u)
  In1/1 -> Demux3/1
  Demux3/1 -> MATLAB Function compute gyroxyz5/1(u)
  Demux3/4 -> MATLAB Function compute gyroxyz3/1(u)

== system ICARO3_orientation_controllo_BIPE/ADIS AHRS2/debias ADIS/Acceleration Detrend /Detrend/Subsystem ==
  In1 : Inport
  Enable : EnablePort
  Constant : Constant  OutDataTypeStr=double
  Discrete-Time Integrator : DiscreteIntegrator  SampleTime=ST  ICPrevOutput=DiscIntNeverNeededParam  ICPrevScaledInput=DiscIntNeverNeededParam
  Discrete-Time Integrator1 : DiscreteIntegrator  InitialCondition=eps  SampleTime=ST  ICPrevOutput=DiscIntNeverNeededParam  ICPrevScaledInput=DiscIntNeverNeededParam
  Product1 : Product  Inputs=*/  SaturateOnIntegerOverflow=on  RndMeth=Zero  InputSameDT=on  OutDataTypeStr=Inherit: Same as first input
  Out2 : Outport
  wires:
  In1/1 -> Discrete-Time Integrator/1
  Discrete-Time Integrator/1 -> Product1/1
  Product1/1 -> Out2/1
  Discrete-Time Integrator1/1 -> Product1/2
  Constant/1 -> Discrete-Time Integrator1/1

== system ICARO3_orientation_controllo_BIPE/ADIS AHRS2/debias ADIS/Acceleration Detrend /Detrend1/Subsystem ==
  In1 : Inport
  Enable : EnablePort
  Constant : Constant
  Discrete-Time Integrator : DiscreteIntegrator  SampleTime=ST  ICPrevOutput=DiscIntNeverNeededParam  ICPrevScaledInput=DiscIntNeverNeededParam
  Discrete-Time Integrator1 : DiscreteIntegrator  InitialCondition=eps  SampleTime=ST  ICPrevOutput=DiscIntNeverNeededParam  ICPrevScaledInput=DiscIntNeverNeededParam
  Product1 : Product  Inputs=*/  SaturateOnIntegerOverflow=on  RndMeth=Zero  InputSameDT=on  OutDataTypeStr=Inherit: Same as first input
  Out2 : Outport
  wires:
  Constant/1 -> Discrete-Time Integrator1/1
  Discrete-Time Integrator1/1 -> Product1/2
  Product1/1 -> Out2/1
  Discrete-Time Integrator/1 -> Product1/1
  In1/1 -> Discrete-Time Integrator/1

== system ICARO3_orientation_controllo_BIPE/ADIS AHRS2/debias ADIS/Acceleration Detrend /Detrend3/Subsystem ==
  In1 : Inport
  Enable : EnablePort
  Constant : Constant
  Discrete-Time Integrator : DiscreteIntegrator  SampleTime=ST  ICPrevOutput=DiscIntNeverNeededParam  ICPrevScaledInput=DiscIntNeverNeededParam
  Discrete-Time Integrator1 : DiscreteIntegrator  InitialCondition=eps  SampleTime=ST  ICPrevOutput=DiscIntNeverNeededParam  ICPrevScaledInput=DiscIntNeverNeededParam
  Product1 : Product  Inputs=*/  SaturateOnIntegerOverflow=on  RndMeth=Zero  InputSameDT=on  OutDataTypeStr=Inherit: Same as first input
  Out2 : Outport
  wires:
  In1/1 -> Discrete-Time Integrator/1
  Discrete-Time Integrator/1 -> Product1/1
  Product1/1 -> Out2/1
  Discrete-Time Integrator1/1 -> Product1/2
  Constant/1 -> Discrete-Time Integrator1/1

== system ICARO3_orientation_controllo_BIPE/ADIS AHRS2/debias ADIS/Gyros Detrend/Detrend/Subsystem ==
  In1 : Inport
  Enable : EnablePort
  Constant : Constant
  Discrete-Time Integrator : DiscreteIntegrator  SampleTime=ST  ICPrevOutput=DiscIntNeverNeededParam  ICPrevScaledInput=DiscIntNeverNeededParam
  Discrete-Time Integrator1 : DiscreteIntegrator  InitialCondition=eps  SampleTime=ST2  ICPrevOutput=DiscIntNeverNeededParam  ICPrevScaledInput=DiscIntNeverNeededParam
  Product1 : Product  Inputs=*/  SaturateOnIntegerOverflow=on  RndMeth=Zero  InputSameDT=on  OutDataTypeStr=Inherit: Same as first input
  Out2 : Outport
  wires:
  Constant/1 -> Discrete-Time Integrator1/1
  Discrete-Time Integrator1/1 -> Product1/2
  Product1/1 -> Out2/1
  Discrete-Time Integrator/1 -> Product1/1
  In1/1 -> Discrete-Time Integrator/1

== system ICARO3_orientation_controllo_BIPE/ADIS AHRS2/debias ADIS/Gyros Detrend/Detrend1/Subsystem ==
  In1 : Inport
  Enable : EnablePort
  Constant : Constant
  Discrete-Time Integrator : DiscreteIntegrator  SampleTime=ST  ICPrevOutput=DiscIntNeverNeededParam  ICPrevScaledInput=DiscIntNeverNeededParam
  Discrete-Time Integrator1 : DiscreteIntegrator  InitialCondition=eps  SampleTime=ST  ICPrevOutput=DiscIntNeverNeededParam  ICPrevScaledInput=DiscIntNeverNeededParam
  Product1 : Product  Inputs=*/  SaturateOnIntegerOverflow=on  RndMeth=Zero  InputSameDT=on  OutDataTypeStr=Inherit: Same as first input
  Out2 : Outport
  wires:
  In1/1 -> Discrete-Time Integrator/1
  Discrete-Time Integrator/1 -> Product1/1
  Product1/1 -> Out2/1
  Discrete-Time Integrator1/1 -> Product1/2
  Constant/1 -> Discrete-Time Integrator1/1

== system ICARO3_orientation_controllo_BIPE/ADIS AHRS2/debias ADIS/Gyros Detrend/Detrend2/Subsystem ==
  In1 : Inport
  Enable : EnablePort
  Constant : Constant
  Discrete-Time Integrator : DiscreteIntegrator  SampleTime=ST  ICPrevOutput=DiscIntNeverNeededParam  ICPrevScaledInput=DiscIntNeverNeededParam
  Discrete-Time Integrator1 : DiscreteIntegrator  InitialCondition=eps  SampleTime=ST  ICPrevOutput=DiscIntNeverNeededParam  ICPrevScaledInput=DiscIntNeverNeededParam
  Product1 : Product  Inputs=*/  SaturateOnIntegerOverflow=on  RndMeth=Zero  InputSameDT=on  OutDataTypeStr=Inherit: Same as first input
  Out2 : Outport
  wires:
  Constant/1 -> Discrete-Time Integrator1/1
  Discrete-Time Integrator1/1 -> Product1/2
  Product1/1 -> Out2/1
  Discrete-Time Integrator/1 -> Product1/1
  In1/1 -> Discrete-Time Integrator/1

== system ICARO3_orientation_controllo_BIPE/ADIS AHRS2/debias ADIS1/Acceleration Detrend /Detrend/Subsystem ==
  In1 : Inport
  Enable : EnablePort
  Constant : Constant  OutDataTypeStr=double
  Discrete-Time Integrator : DiscreteIntegrator  SampleTime=ST  ICPrevOutput=DiscIntNeverNeededParam  ICPrevScaledInput=DiscIntNeverNeededParam
  Discrete-Time Integrator1 : DiscreteIntegrator  InitialCondition=eps  SampleTime=ST  ICPrevOutput=DiscIntNeverNeededParam  ICPrevScaledInput=DiscIntNeverNeededParam
  Product1 : Product  Inputs=*/  OutDataTypeStr=Inherit: Inherit via back propagation  SaturateOnIntegerOverflow=on  RndMeth=Zero
  Out2 : Outport
  wires:
  In1/1 -> Discrete-Time Integrator/1
  Discrete-Time Integrator/1 -> Product1/1
  Product1/1 -> Out2/1
  Discrete-Time Integrator1/1 -> Product1/2
  Constant/1 -> Discrete-Time Integrator1/1

== system ICARO3_orientation_controllo_BIPE/ADIS AHRS2/debias ADIS1/Acceleration Detrend /Detrend1/Subsystem ==
  In1 : Inport
  Enable : EnablePort
  Constant : Constant
  Discrete-Time Integrator : DiscreteIntegrator  SampleTime=ST  ICPrevOutput=DiscIntNeverNeededParam  ICPrevScaledInput=DiscIntNeverNeededParam
  Discrete-Time Integrator1 : DiscreteIntegrator  InitialCondition=eps  SampleTime=ST  ICPrevOutput=DiscIntNeverNeededParam  ICPrevScaledInput=DiscIntNeverNeededParam
  Product1 : Product  Inputs=*/  OutDataTypeStr=Inherit: Inherit via back propagation  SaturateOnIntegerOverflow=on  RndMeth=Zero
  Out2 : Outport
  wires:
  Constant/1 -> Discrete-Time Integrator1/1
  Discrete-Time Integrator1/1 -> Product1/2
  Product1/1 -> Out2/1
  Discrete-Time Integrator/1 -> Product1/1
  In1/1 -> Discrete-Time Integrator/1

== system ICARO3_orientation_controllo_BIPE/ADIS AHRS2/debias ADIS1/Acceleration Detrend /Detrend3/Subsystem ==
  In1 : Inport
  Enable : EnablePort
  Constant : Constant  OutDataTypeStr=single
  Discrete-Time Integrator : DiscreteIntegrator  SampleTime=ST  ICPrevOutput=DiscIntNeverNeededParam  ICPrevScaledInput=DiscIntNeverNeededParam
  Discrete-Time Integrator1 : DiscreteIntegrator  InitialCondition=eps  SampleTime=ST  ICPrevOutput=DiscIntNeverNeededParam  ICPrevScaledInput=DiscIntNeverNeededParam
  Product1 : Product  Inputs=*/  OutDataTypeStr=Inherit: Inherit via back propagation  SaturateOnIntegerOverflow=on  RndMeth=Zero  InputSameDT=on
  Out2 : Outport
  wires:
  In1/1 -> Discrete-Time Integrator/1
  Discrete-Time Integrator/1 -> Product1/1
  Product1/1 -> Out2/1
  Discrete-Time Integrator1/1 -> Product1/2
  Constant/1 -> Discrete-Time Integrator1/1

== system ICARO3_orientation_controllo_BIPE/ADIS AHRS2/debias ADIS1/Acceleration Detrend 1/Detrend/Subsystem ==
  In1 : Inport
  Enable : EnablePort
  Constant : Constant  OutDataTypeStr=double
  Discrete-Time Integrator : DiscreteIntegrator  SampleTime=ST  ICPrevOutput=DiscIntNeverNeededParam  ICPrevScaledInput=DiscIntNeverNeededParam
  Discrete-Time Integrator1 : DiscreteIntegrator  InitialCondition=eps  SampleTime=ST  ICPrevOutput=DiscIntNeverNeededParam  ICPrevScaledInput=DiscIntNeverNeededParam
  Product1 : Product  Inputs=*/  SaturateOnIntegerOverflow=on  RndMeth=Zero  InputSameDT=on  OutDataTypeStr=Inherit: Same as first input
  Out2 : Outport
  wires:
  In1/1 -> Discrete-Time Integrator/1
  Discrete-Time Integrator/1 -> Product1/1
  Product1/1 -> Out2/1
  Discrete-Time Integrator1/1 -> Product1/2
  Constant/1 -> Discrete-Time Integrator1/1

== system ICARO3_orientation_controllo_BIPE/ADIS AHRS2/debias ADIS1/Acceleration Detrend 1/Detrend1/Subsystem ==
  In1 : Inport
  Enable : EnablePort
  Constant : Constant
  Discrete-Time Integrator : DiscreteIntegrator  SampleTime=ST  ICPrevOutput=DiscIntNeverNeededParam  ICPrevScaledInput=DiscIntNeverNeededParam
  Discrete-Time Integrator1 : DiscreteIntegrator  InitialCondition=eps  SampleTime=ST  ICPrevOutput=DiscIntNeverNeededParam  ICPrevScaledInput=DiscIntNeverNeededParam
  Product1 : Product  Inputs=*/  SaturateOnIntegerOverflow=on  RndMeth=Zero  InputSameDT=on  OutDataTypeStr=Inherit: Same as first input
  Out2 : Outport
  wires:
  Constant/1 -> Discrete-Time Integrator1/1
  Discrete-Time Integrator1/1 -> Product1/2
  Product1/1 -> Out2/1
  Discrete-Time Integrator/1 -> Product1/1
  In1/1 -> Discrete-Time Integrator/1

== system ICARO3_orientation_controllo_BIPE/ADIS AHRS2/debias ADIS1/Acceleration Detrend 1/Detrend3/Subsystem ==
  In1 : Inport
  Enable : EnablePort
  Constant : Constant
  Discrete-Time Integrator : DiscreteIntegrator  SampleTime=ST  ICPrevOutput=DiscIntNeverNeededParam  ICPrevScaledInput=DiscIntNeverNeededParam
  Discrete-Time Integrator1 : DiscreteIntegrator  InitialCondition=eps  SampleTime=ST  ICPrevOutput=DiscIntNeverNeededParam  ICPrevScaledInput=DiscIntNeverNeededParam
  Product1 : Product  Inputs=*/  SampleTime=0.01  SaturateOnIntegerOverflow=on  RndMeth=Zero  InputSameDT=on  OutDataTypeStr=Inherit: Same as first input
  Out2 : Outport
  wires:
  In1/1 -> Discrete-Time Integrator/1
  Discrete-Time Integrator/1 -> Product1/1
  Product1/1 -> Out2/1
  Discrete-Time Integrator1/1 -> Product1/2
  Constant/1 -> Discrete-Time Integrator1/1

== system ICARO3_orientation_controllo_BIPE/ADIS AHRS2/debias ADIS1/Gyros Detrend/Detrend/Subsystem ==
  In1 : Inport
  Enable : EnablePort
  Constant : Constant  OutDataTypeStr=single
  Discrete-Time Integrator : DiscreteIntegrator  SampleTime=ST  ICPrevOutput=DiscIntNeverNeededParam  ICPrevScaledInput=DiscIntNeverNeededParam
  Discrete-Time Integrator1 : DiscreteIntegrator  InitialCondition=eps  SampleTime=ST2  ICPrevOutput=DiscIntNeverNeededParam  ICPrevScaledInput=DiscIntNeverNeededParam
  Product1 : Product  Inputs=*/  SaturateOnIntegerOverflow=on  RndMeth=Zero  InputSameDT=on  OutDataTypeStr=Inherit: Same as first input
  Out2 : Outport
  wires:
  Constant/1 -> Discrete-Time Integrator1/1
  Discrete-Time Integrator1/1 -> Product1/2
  Product1/1 -> Out2/1
  Discrete-Time Integrator/1 -> Product1/1
  In1/1 -> Discrete-Time Integrator/1

== system ICARO3_orientation_controllo_BIPE/ADIS AHRS2/debias ADIS1/Gyros Detrend/Detrend1/Subsystem ==
  In1 : Inport
  Enable : EnablePort
  Constant : Constant
  Data Type Conversion mx3 : DataTypeConversion  OutDataTypeStr=single  RndMeth=Round  SaturateOnIntegerOverflow=on
  Discrete-Time Integrator : DiscreteIntegrator  SampleTime=ST  ICPrevOutput=DiscIntNeverNeededParam  ICPrevScaledInput=DiscIntNeverNeededParam
  Discrete-Time Integrator1 : DiscreteIntegrator  InitialCondition=eps  SampleTime=ST  ICPrevOutput=DiscIntNeverNeededParam  ICPrevScaledInput=DiscIntNeverNeededParam
  Product1 : Product  Inputs=*/  SaturateOnIntegerOverflow=on  RndMeth=Zero  InputSameDT=on  OutDataTypeStr=Inherit: Same as first input
  Out2 : Outport
  wires:
  In1/1 -> Discrete-Time Integrator/1
  Discrete-Time Integrator/1 -> Product1/1
  Product1/1 -> Out2/1
  Discrete-Time Integrator1/1 -> Data Type Conversion mx3/1
  Constant/1 -> Discrete-Time Integrator1/1
  Data Type Conversion mx3/1 -> Product1/2

== system ICARO3_orientation_controllo_BIPE/ADIS AHRS2/debias ADIS1/Gyros Detrend/Detrend2/Subsystem ==
  In1 : Inport
  Enable : EnablePort
  Constant : Constant
  Data Type Conversion mx3 : DataTypeConversion  OutDataTypeStr=single  RndMeth=Round  SaturateOnIntegerOverflow=on
  Discrete-Time Integrator : DiscreteIntegrator  SampleTime=ST  ICPrevOutput=DiscIntNeverNeededParam  ICPrevScaledInput=DiscIntNeverNeededParam
  Discrete-Time Integrator1 : DiscreteIntegrator  InitialCondition=eps  SampleTime=ST  ICPrevOutput=DiscIntNeverNeededParam  ICPrevScaledInput=DiscIntNeverNeededParam
  Product1 : Product  Inputs=*/  SaturateOnIntegerOverflow=on  RndMeth=Zero  InputSameDT=on  OutDataTypeStr=Inherit: Same as first input
  Out2 : Outport
  wires:
  Constant/1 -> Discrete-Time Integrator1/1
  Discrete-Time Integrator1/1 -> Data Type Conversion mx3/1
  Product1/1 -> Out2/1
  Discrete-Time Integrator/1 -> Product1/1
  In1/1 -> Discrete-Time Integrator/1
  Data Type Conversion mx3/1 -> Product1/2

== system ICARO3_orientation_controllo_BIPE/SS AHRS/debias SS/Acceleration Detrend /Detrend/Subsystem ==
  In1 : Inport
  Enable : EnablePort
  Constant : Constant  OutDataTypeStr=double
  Discrete-Time Integrator : DiscreteIntegrator  SampleTime=ST  ICPrevOutput=DiscIntNeverNeededParam  ICPrevScaledInput=DiscIntNeverNeededParam
  Discrete-Time Integrator1 : DiscreteIntegrator  InitialCondition=eps  SampleTime=ST  ICPrevOutput=DiscIntNeverNeededParam  ICPrevScaledInput=DiscIntNeverNeededParam
  Product1 : Product  Inputs=*/  SaturateOnIntegerOverflow=on  RndMeth=Zero  InputSameDT=on  OutDataTypeStr=Inherit: Same as first input
  Out2 : Outport
  wires:
  Constant/1 -> Discrete-Time Integrator1/1
  Discrete-Time Integrator1/1 -> Product1/2
  Product1/1 -> Out2/1
  Discrete-Time Integrator/1 -> Product1/1
  In1/1 -> Discrete-Time Integrator/1

== system ICARO3_orientation_controllo_BIPE/SS AHRS/debias SS/Acceleration Detrend /Detrend1/Subsystem ==
  In1 : Inport
  Enable : EnablePort
  Constant : Constant
  Discrete-Time Integrator : DiscreteIntegrator  SampleTime=ST  ICPrevOutput=DiscIntNeverNeededParam  ICPrevScaledInput=DiscIntNeverNeededParam
  Discrete-Time Integrator1 : DiscreteIntegrator  InitialCondition=eps  SampleTime=ST  ICPrevOutput=DiscIntNeverNeededParam  ICPrevScaledInput=DiscIntNeverNeededParam
  Product1 : Product  Inputs=*/  SaturateOnIntegerOverflow=on  RndMeth=Zero  InputSameDT=on  OutDataTypeStr=Inherit: Same as first input
  Out2 : Outport
  wires:
  In1/1 -> Discrete-Time Integrator/1
  Discrete-Time Integrator/1 -> Product1/1
  Product1/1 -> Out2/1
  Discrete-Time Integrator1/1 -> Product1/2
  Constant/1 -> Discrete-Time Integrator1/1
